simulink model "MINE"  (R2022b)
settings: Solver=ode45  StartTime=0.0  StopTime=10.0  MaxStep=.001  RelTol=1e-3  AbsTol=1e-6
values from neighbouring files (symbols this model uses):
  A = [a11       0        0      a14       0        0       0     a22        0        0       0      a26       0       0        0        1       0        0     a41       0      a43      a44     a45        0       0       0        0        0       0        1       0     a62      a63        0     a65      a66]    [HW6_MINE.m]
  B = [b11     0       0   b22       0     0       0     0       0     0       0     0]    [HW6_MINE.m]
  C = [0 0 1 0 0 0    0 0 0 0 1 0]    [HW6_MINE.m]
  D = [0 0    0 0]    [HW6_MINE.m]
  Klag = 1    [HW6_MINE.m]
  lagpole = 1    [HW6_MINE.m]
  lagzero = 0.991    [HW6_MINE.m]
  leadpole = 0.2    [HW6_MINE.m]
  leadzero = 0.46415    [HW6_MINE.m]
  sensor_delay = inptdf(['\nEnter theta2 sensor delay time (sec) [' delaytxt ']'],sensor_delay)    [HW6_MINE.m]
  sensor_gain = inptdf(['\nEnter theta2 sensor gain (dimensionless) [' gaintxt ']'],sensor_gain)    [HW6_MINE.m]
undefined symbols (not defined in the file or in its folder): Klead, theta2ref, Ts
settings Model: Creator=mcb  LastModifiedBy=ROG
settings SolverCC: AutoScaleAbsTol=off  AlgebraicLoopSolver=TrustRegion
settings DataIOCC: SaveFormat=Array  SignalLoggingSaveFormat=ModelDataLogs  SaveOutput=off  SignalLogging=off  DSMLogging=off  VisualizeSimOutput=off  SaveTime=off  ReturnWorkspaceOutputs=off  TimeSaveName=t_sim  OutputSaveName=y_sim  SignalLoggingName=sigsOut
settings OptimizationCC: BooleanDataType=off  LifeSpan=inf
settings DebuggingCC: SaveWithParameterizedLinksMsg=none  UnderspecifiedInitializationDetection=Classic  MergeDetectMultiDrivingBlocksExec=none  SignalResolutionControl=TryResolveAllWithWarning  MultiTaskDSMMsg=warning  MultiTaskCondExecSysMsg=none  UnconnectedInputMsg=warning  UnconnectedOutputMsg=warning  UnconnectedLineMsg=warning  SFUnexpectedBacktrackingDiag=warning  SFNoUnconditionalDefaultTransitionDiag=warning  SFExecutionAtInitializationDiag=none  SFMachineParentedDataDiag=warning  ArithmeticOperatorsInVariantConditions=warning
settings HardwareCC: ProdBitPerPointer=32  ProdBitPerSizeT=32  ProdBitPerPtrDiffT=32  ProdLargestAtomicFloat=None  ProdIntDivRoundTo=Undefined  ProdEndianess=Unspecified  ProdWordSize=32  ProdHWDeviceType=32-bit Generic  TargetUnknown=on
settings ModelReferenceCC: PropagateSignalLabelsOutOfModel=off
settings SFSimCC: SimUseLocalCustomCode=off  CustomCodeUndefinedFunction=UseInterfaceOnly
settings RTWCC: TemplateMakefile=grt_vc.tmf  RTWUseLocalCustomCode=off
settings CodeAppCC: StateflowObjectComments=on
settings GRTTargetCC: TargetLangStandard=C89/C90 (ANSI)  CombineOutputUpdateFcns=off  GRTInterface=on
settings ConfigComp: CovMetricSettings=dw  CovSaveCumulativeToWorkspaceVar=on  CovSaveSingleToWorkspaceVar=on  CovExternalEMLEnable=off  CovSFcnEnable=off

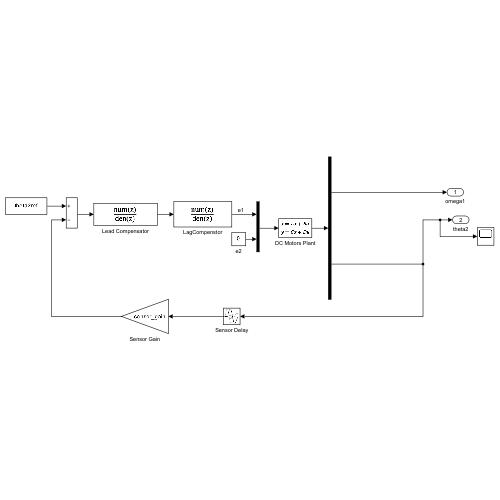
[thumbnail: Simulink's stored preview of the top-level diagram]
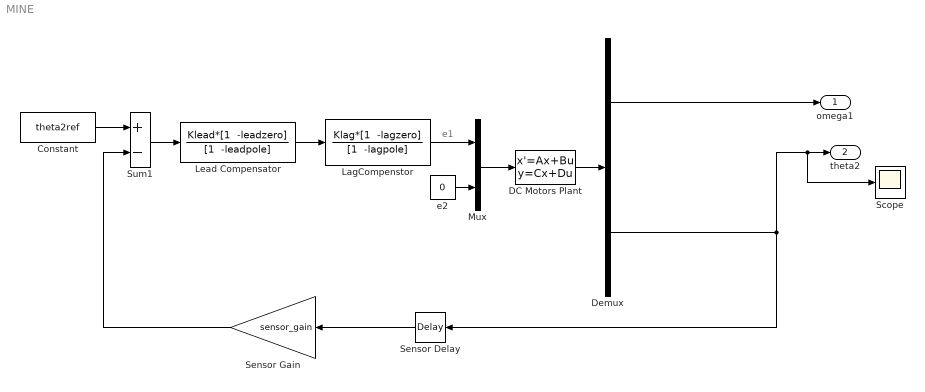
== system MINE ==
  note: e1
  Constant : Constant  Value=theta2ref
  DC Motors Plant : StateSpace  A=A  B=B  C=C  D=D  InitialCondition=0
  Demux : Demux  Outputs=2
      settings: DisplayOption=none
  LagCompenstor : DiscreteTransferFcn  Numerator="Klag*[1  -lagzero]"  Denominator="[1  -lagpole]"  SampleTime=Ts
  Lead Compensator : DiscreteTransferFcn  Numerator="Klead*[1  -leadzero]"  Denominator="[1  -leadpole]"  SampleTime=Ts
  Mux : Mux  Inputs=2
  Scope : Scope
  Sensor Delay : TransportDelay  DelayTime=sensor_delay
  Sensor Gain : Gain  Gain=sensor_gain  SaturateOnIntegerOverflow=on  OutDataTypeStr=Inherit: Same as input  ParamDataTypeStr=Inherit: Same as input
  Sum1 : Sum  Inputs=+-  InputSameDT=on  SaturateOnIntegerOverflow=on  OutDataTypeStr=Inherit: Same as first input
  e2 : Constant  Value=0
  omega1 : Outport
  theta2 : Outport  Port=2
  wires:
  Constant/1 -> Sum1/1
  Lead Compensator/1 -> LagCompenstor/1
  LagCompenstor/1 -> Mux/1
  Mux/1 -> DC Motors Plant/1
  e2/1 -> Mux/2
  DC Motors Plant/1 -> Demux/1
  Demux/2 -> Scope/1, theta2/1, Sensor Delay/1
  Sum1/1 -> Lead Compensator/1
  Demux/1 -> omega1/1
  Sensor Delay/1 -> Sensor Gain/1
  Sensor Gain/1 -> Sum1/2
